simulink model "equalizer_IIR"  (R2019b)
settings: Solver=VariableStepAuto  StartTime=0.0  StopTime=10.0  RelTol=1e-3
libraries: dsparch4 x5, dspmathops x5, dspsnks4 x1, dspvision x1
settings Model: Creator=demid  LastModifiedBy=demid

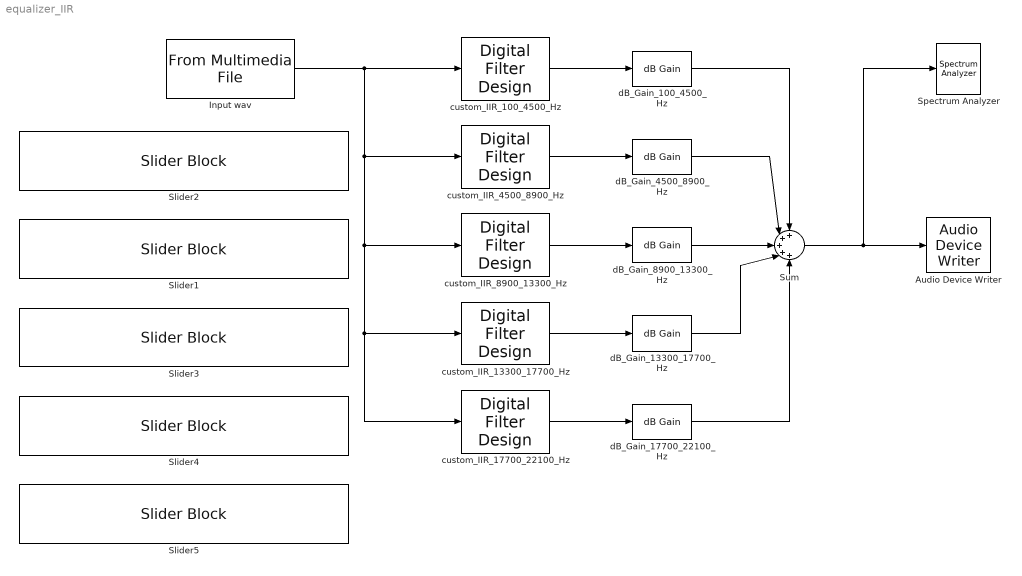
== system equalizer_IIR ==
  Audio Device Writer : dspsnks4/Audio Device Writer  Driver=CoreAudio  Device=Динамики �MacBook Pro�  InheritSampleRate=on  SampleRate=44100  BitDepth=16-bit integer  BufferSize=4096  NumBuffers=10  DefaultOutputChannelMapping=on  OutputChannelMapping=1:2  OutputNumUnderrunSamples=off  DriverIdx=5  DeviceWarnFlag=''
  Input wav : dspvision/From Multimedia File  inputFilename=/Users/demid/repos/IU4-22M/Leo_MatLab/Songs/Red_alert_3_USSR_anthem.wav  readRange=[1 Inf]  loop=on  numPlays=inf  outputStreams=Audio only  videoDataType=single  audioDataType=double  inheritSampleTime=on  userDefinedSampleTime=1/30  noAudioOutput=off  isIntensityVideo=off  fourcc=RGB  colorVideoFormat=Separate color signals  outputEOF=off  dataOrg=Column-major  audioFrameSize=1024  computeAudioFrameSize=off  outSamplingMode=Sample based
      settings: SourceProductName=DSP System Toolbox  SourceProductBaseCode=DS
  Slider{1..5} (5 alike) : SliderBlock  ScaleMin=-100
  Spectrum Analyzer : SpectrumAnalyzer
  Sum : Sum  Inputs=+++++
  custom_IIR_100_4500_Hz : dsparch4/Digital Filter Design  mwdsp_browser_bugfix_var=off
  custom_IIR_13300_17700_Hz : dsparch4/Digital Filter Design  mwdsp_browser_bugfix_var=off
  custom_IIR_17700_22100_Hz : dsparch4/Digital Filter Design  mwdsp_browser_bugfix_var=off
  custom_IIR_4500_8900_Hz : dsparch4/Digital Filter Design  mwdsp_browser_bugfix_var=off
  custom_IIR_8900_13300_Hz : dsparch4/Digital Filter Design  mwdsp_browser_bugfix_var=off
  dB_Gain_100_4500_Hz : dspmathops/dB Gain  dB=7.315613026819932  intype=Amplitude
      settings: SourceProductName=DSP System Toolbox  SourceProductBaseCode=DS
  dB_Gain_13300_17700_Hz : dspmathops/dB Gain  dB=11.147030651341  intype=Amplitude
      settings: SourceProductName=DSP System Toolbox  SourceProductBaseCode=DS
  dB_Gain_17700_22100_Hz : dspmathops/dB Gain  dB=12.67959770114942  intype=Amplitude
      settings: SourceProductName=DSP System Toolbox  SourceProductBaseCode=DS
  dB_Gain_4500_8900_Hz : dspmathops/dB Gain  dB=7.315613026819932  intype=Amplitude
      settings: SourceProductName=DSP System Toolbox  SourceProductBaseCode=DS
  dB_Gain_8900_13300_Hz : dspmathops/dB Gain  dB=8.081896551724128  intype=Amplitude
      settings: SourceProductName=DSP System Toolbox  SourceProductBaseCode=DS
  wires:
  Input wav/1 -> custom_IIR_4500_8900_Hz/1, custom_IIR_8900_13300_Hz/1, custom_IIR_13300_17700_Hz/1, custom_IIR_17700_22100_Hz/1, custom_IIR_100_4500_Hz/1
  custom_IIR_100_4500_Hz/1 -> dB_Gain_100_4500_Hz/1
  custom_IIR_4500_8900_Hz/1 -> dB_Gain_4500_8900_Hz/1
  custom_IIR_8900_13300_Hz/1 -> dB_Gain_8900_13300_Hz/1
  custom_IIR_13300_17700_Hz/1 -> dB_Gain_13300_17700_Hz/1
  custom_IIR_17700_22100_Hz/1 -> dB_Gain_17700_22100_Hz/1
  dB_Gain_8900_13300_Hz/1 -> Sum/3
  dB_Gain_4500_8900_Hz/1 -> Sum/2
  dB_Gain_100_4500_Hz/1 -> Sum/1
  dB_Gain_13300_17700_Hz/1 -> Sum/4
  dB_Gain_17700_22100_Hz/1 -> Sum/5
  Sum/1 -> Spectrum Analyzer/1, Audio Device Writer/1
